simulink model "commhdlQPSKTxRxLoopback"  (R2025b)
settings: Solver=FixedStepDiscrete  StartTime=0.0  StopTime=stopTime  RelTol=1e-3
PostLoadFcn:
  | hScopeConfig = get_param([gcs '/Receiver/QPSK Rx/Frequency and Time Synchronizer/Symbol Synchronizer/No HDL/QPSK Receiver Eye Diagram'],'ScopeConfiguration');
  | 
  | hScopeConfig.OpenAtSimulationStart = false;
  | hScopeConfig.Visible = false;
  | SamplesPerSymbol = 4;
  | %UpsamplesRx = 1;
  | clear hScopeConfig
InitFcn:
  | commhdlQPSKTxRxModelInit;
  | % Rate bridge: ADRV9002/Jupiter radio runs at 15.36 MHz = 2x the 7.68 MHz
  | % (4 samples/symbol @ Rsym=1.92 MHz) the QPSK Rx requires. The deployed
  | % Receiver must downsample the ADC stream by 2. UpsamplesRx=1 fed the QPSK
  | % Rx 8 sps (2x-upsampled) and broke symbol sync / the loopback bit check.
  | UpsamplesRx = 1;   %% T8 RATE FIX: rail 15.36e6 == ADC bus rate,
  | %% no ingress decimation (was 2 when the rail sat on the 7.68e6 rung)
  | UpsamplesTx = 1;
  | clear simTimingOffset;
StopFcn:
  | if exist('simTimingOffset','var')
  |   disp('Simulation completed');
  |   %QPSKTxRxVerification;
  | end
values from neighbouring files (symbols this model uses):
  Config = commhdlQPSKTxRxParameters    [commhdlQPSKTxRxModelInit.m]
  Rsym = eval(get_param(qpskFindTxInputData(gcs),'Rsym'))    [commhdlQPSKTxRxModelInit.m]
undefined symbols (not defined in the file or in its folder): Add, fsym, randsrc, RandStream, Shift
libraries: hdlsllib x143, simulink x45, dspsigops x34, dsphdlfiltering2 x6, dsphdlsigops2 x4, dsphdlmathfun2 x4, commdigbbndpm3 x4, dspmlti4 x2, commchan3 x1, commrflib2 x1, commcnvcod2 x1
(part 7 of 8)

== system commhdlQPSKTxRxLoopback/TxRxComposite/Receiver/QPSK Rx/Frequency and Time Synchronizer/Preamble Detector/FIFO/Validate Input Push Pop ==
  rst : Inport
  push : Inport  Port=2
  pop : Inport  Port=3
  Compare To Constant : hdlsllib/Logic and Bit Operations/Compare To Constant  relop===  const=0  OutDataTypeStr=boolean
  Compare To Constant1 : hdlsllib/Logic and Bit Operations/Compare To Constant  relop===  const=fifoSize  OutDataTypeStr=boolean
  Constant : Constant  Value=true  SampleTime=-1
  Constant1 : Constant  Value=false  SampleTime=-1
  Delay : Delay  DelayLength=1
  Logical Operator1 : Logic  Operator=XOR  AllPortsSameDT=off  OutDataTypeStr=boolean
  Logical Operator2 : Logic  Operator=NOT  AllPortsSameDT=off  OutDataTypeStr=boolean
  Logical Operator{3..5,7,9} (5 alike) : Logic  AllPortsSameDT=off  OutDataTypeStr=boolean
  Logical Operator6 : Logic  Operator=NOT  AllPortsSameDT=off  OutDataTypeStr=boolean
  Logical Operator8 : Logic  Operator=NOT  AllPortsSameDT=off  OutDataTypeStr=boolean
  MATLAB Function : MATLAB Function  TreatAsAtomicUnit=on  mask{initVal=0, countToVal=fifoSize}
      mask prompts: initVal "Initial value:"; countToVal "Count to value:"
  No HDL : Subsystem
  Switch : Switch  Criteria=u2 ~= 0  SaturateOnIntegerOverflow=off  InputSameDT=off
  valid push : Outport
  valid pop : Outport  Port=2
  numEntries : Outport  Port=3
  wires:
  Delay/1 -> Compare To Constant/1, numEntries/1, Compare To Constant1/1
  rst/1 -> MATLAB Function/1(rst)
  Compare To Constant/1 -> Logical Operator3/1
  pop/1 -> Logical Operator7/1, Logical Operator3/2
  Switch/1 -> MATLAB Function/3(dir)
  MATLAB Function/1(count) -> Delay/1
  Constant1/1 -> Switch/1
  Logical Operator3/1 -> Logical Operator6/1, No HDL/2(popEmptyFIFO)  "pop on empty FIFO"
  Logical Operator4/1 -> Logical Operator2/1, No HDL/1(pushFullFIFO)  "push on full FIFO"
  Constant/1 -> Switch/3
  Compare To Constant1/1 -> Logical Operator4/2
  Logical Operator7/1 -> Logical Operator1/2, Logical Operator8/1, valid pop/1, Switch/2
  Logical Operator6/1 -> Logical Operator7/2
  Logical Operator1/1 -> MATLAB Function/2(enb)
  push/1 -> Logical Operator9/1, Logical Operator5/1
  Logical Operator8/1 -> Logical Operator5/2
  Logical Operator5/1 -> Logical Operator4/1
  Logical Operator2/1 -> Logical Operator9/2
  Logical Operator9/1 -> valid push/1, Logical Operator1/1

== system commhdlQPSKTxRxLoopback/TxRxComposite/Receiver/QPSK Rx/Frequency and Time Synchronizer/Preamble Detector/Timing Adjust/No HDL ==
  note: This subsystem generates variables required for QPSKRxVerification for validation
  validIn : Inport
  timingOffset : Inport  Port=2
  syncPulse : Inport  Port=3
  Compare To Constant : simulink/Logic and Bit Operations/Compare To Constant  relop===  const=0  OutDataTypeStr=boolean
  Delay : Delay  DelayLength=4
  Delay1 : Delay  DelayLength=4
  Frame Counter : hdlsllib/Sources/HDL Counter  CountType=Free running  CountInit=0  CountStep=1  CountMax=bitsPerPacket/2 - 1  CountFromType=Initial value  CountFrom=0  CountResetPort=off  CountLoadPort=off  CountEnbPort=on  CountDirPort=off  CountHitOutputPort=off  CountDataType=Unsigned  CountWordLen=32  CountFracLen=0  CountSampTime=1
  Logical Operator : Logic  AllPortsSameDT=off  OutDataTypeStr=boolean
  No HDL : Subsystem
  No HDL1 : Subsystem
  Symbol Counter : hdlsllib/Sources/HDL Counter  CountType=Count limited  CountInit=0  CountStep=1  CountMax=bitsPerPacket/2 - 1  CountFromType=Initial value  CountFrom=0  CountResetPort=off  CountLoadPort=off  CountEnbPort=on  CountDirPort=off  CountHitOutputPort=off  CountDataType=Unsigned  CountWordLen=nextpow2(bitsPerPacket/2 - 1)  CountFracLen=0  CountSampTime=1
  Unit Delay Enabled Synchronous : hdlsllib/Discrete/Unit Delay Enabled Synchronous  InitialCondition=0.0  SampleTime=-1
  wires:
  Delay1/1 -> No HDL/1(timingOffset)
  Delay/1 -> No HDL1/Enable, No HDL/Enable
  Unit Delay Enabled Synchronous/1 -> No HDL1/1(frameNumber)
  syncPulse/1 -> Delay/1
  Frame Counter/1 -> Unit Delay Enabled Synchronous/1
  Compare To Constant/1 -> Logical Operator/1
  Logical Operator/1 -> Frame Counter/1, Unit Delay Enabled Synchronous/2
  Symbol Counter/1 -> Compare To Constant/1
  validIn/1 -> Symbol Counter/1, Logical Operator/2
  timingOffset/1 -> Delay1/1

== system commhdlQPSKTxRxLoopback/TxRxComposite/Receiver/QPSK Rx/Frequency and Time Synchronizer/Symbol Synchronizer/Gardner TED/GTED ==
  In1 : Inport
  Add : Sum
  Add1 : Sum  Inputs=+-
  Add2 : Sum  Inputs=+-
  Complex to Real-Imag : ComplexToRealImag
  Delay{,1,4..5} (4 alike) : Delay  DelayLength=1
  Delay{9..10,12..13} (4 alike) : Delay
  Delay11 : Delay  DelayLength=4
  Delay{2..3,6..7} (4 alike) : Delay  DelayLength=3
  Delay8 : Delay  DelayLength=4
  Product : Product
  Product1 : Product
  Out1 : Outport
  wires:
  Delay13/1 -> Add/2
  Delay12/1 -> Product1/2
  Delay11/1 -> Product1/1
  Delay10/1 -> Add/1
  Delay9/1 -> Product/2
  Delay8/1 -> Product/1
  Complex to Real-Imag/2 -> Delay4/1, Add2/2
  Delay7/1 -> Add2/1
  Delay4/1 -> Delay5/1
  Delay6/1 -> Delay7/1
  Add2/1 -> Delay12/1
  Delay5/1 -> Delay6/1, Delay11/1
  Delay1/1 -> Delay8/1, Delay2/1
  Add1/1 -> Delay9/1
  Delay2/1 -> Delay3/1
  Delay/1 -> Delay1/1
  Delay3/1 -> Add1/1
  Complex to Real-Imag/1 -> Delay/1, Add1/2
  In1/1 -> Complex to Real-Imag/1
  Add/1 -> Out1/1
  Product1/1 -> Delay13/1
  Product/1 -> Delay10/1

== system commhdlQPSKTxRxLoopback/TxRxComposite/Receiver/QPSK Rx/Frequency and Time Synchronizer/Symbol Synchronizer/No HDL/No HDL ==
  data : Inport
  Enable : EnablePort
  Data Type Conversion : DataTypeConversion  OutDataTypeStr=double  SaturateOnIntegerOverflow=off  RndMeth=Floor
  wires:
  data/1 -> Data Type Conversion/1
  Data Type Conversion/1 -> ?

== system commhdlQPSKTxRxLoopback/TxRxComposite/Receiver/QPSK Rx/Frequency and Time Synchronizer/Symbol Synchronizer/Rate Handle/FIFO ==
  in : Inport
  push : Inport  Port=2
  pop : Inport  Port=3
  reset : Inport  Port=4
  Delay1 : Delay  DelayLength=1
  Pop Counter : hdlsllib/Sources/HDL Counter  CountType=Count limited  CountInit=0  CountStep=1  CountMax=fifoSize -1  CountFromType=Initial value  CountFrom=0  CountResetPort=on  CountLoadPort=off  CountEnbPort=on  CountDirPort=off  CountHitOutputPort=off  CountDataType=Unsigned  CountWordLen=nextpow2(fifoSize)  CountFracLen=0  CountSampTime=1
  Push Counter : hdlsllib/Sources/HDL Counter  CountType=Count limited  CountInit=0  CountStep=1  CountMax=fifoSize -1  CountFromType=Initial value  CountFrom=0  CountResetPort=on  CountLoadPort=off  CountEnbPort=on  CountDirPort=off  CountHitOutputPort=off  CountDataType=Unsigned  CountWordLen=nextpow2(fifoSize)  CountFracLen=0  CountSampTime=1
  Simple Dual Port RAM : hdlsllib/HDL RAMs/Simple Dual Port RAM  ram_size=nextpow2(fifoSize)
  Validate Input Push Pop : Subsystem
  out : Outport
  numEntries : Outport  Port=2
  validPop : Outport  Port=3
  wires:
  Validate Input Push Pop/3(numEntries) -> numEntries/1
  Simple Dual Port RAM/1 -> out/1
  Push Counter/1 -> Simple Dual Port RAM/2
  Pop Counter/1 -> Simple Dual Port RAM/4
  push/1 -> Validate Input Push Pop/2(push)
  pop/1 -> Validate Input Push Pop/3(pop)
  Validate Input Push Pop/1(valid push) -> Simple Dual Port RAM/3, Push Counter/2
  Validate Input Push Pop/2(valid pop) -> validPop/1, Pop Counter/2
  reset/1 -> Delay1/1, Validate Input Push Pop/1(rst)
  in/1 -> Simple Dual Port RAM/1
  Delay1/1 -> Pop Counter/1, Push Counter/1

== system commhdlQPSKTxRxLoopback/TxRxComposite/Transmitter/QPSK Tx/Bit Packetizer/Data Bits FIFO/No HDL/No HDL ==
  push : Inport
  full : Inport  Port=2
  ncount : Inport  Port=3
  empty : Inport  Port=4
  pop : Inport  Port=5
  Assertion : Assertion
  Assertion1 : Assertion
  Display : Display
  Logical Operator : Logic  Operator=NAND  AllPortsSameDT=off  OutDataTypeStr=boolean
  Logical Operator1 : Logic  Operator=NAND  AllPortsSameDT=off  OutDataTypeStr=boolean
  wires:
  push/1 -> Logical Operator/1
  empty/1 -> Logical Operator1/1
  full/1 -> Logical Operator/2
  pop/1 -> Logical Operator1/2
  Logical Operator/1 -> Assertion/1
  ncount/1 -> Display/1
  Logical Operator1/1 -> Assertion1/1

== system commhdlQPSKTxRxLoopback/Receiver/QPSK Rx/Frequency and Time Synchronizer/Symbol Synchronizer/Rate Handle/FIFO/Validate Input Push Pop/No HDL ==
  pushFullFIFO : Inport
  popEmptyFIFO : Inport  Port=2
  Constant2 : Constant  Value=pushFullDiag  SampleTime=-1
  Constant3 : Constant  Value=popEmptyDiag  SampleTime=-1
  MATLAB Function : MATLAB Function  TreatAsAtomicUnit=on
  wires:
  Constant2/1 -> MATLAB Function/1(pushFullDiag)
  Constant3/1 -> MATLAB Function/2(popEmptyDiag)
  popEmptyFIFO/1 -> MATLAB Function/4(popEmpty)
  pushFullFIFO/1 -> MATLAB Function/3(pushFull)

== system commhdlQPSKTxRxLoopback/TxRxComposite/Receiver/QPSK Rx/Frequency and Time Synchronizer/Coarse Frequency Compensator/Coarse Frequency Estimator/Integrator/Reset Generator ==
  validIn : Inport
  Compare To Constant : simulink/Logic and Bit Operations/Compare To Constant  relop===  const=integAvgLen  OutDataTypeStr=boolean
  Delay1 : Delay  DelayLength=1
  Delay5 : Delay  DelayLength=1
  HDL Counter : hdlsllib/Sources/HDL Counter  CountType=Count limited  CountInit=0  CountStep=1  CountMax=integAvgLen  CountFromType=Initial value  CountFrom=0  CountResetPort=off  CountLoadPort=off  CountEnbPort=on  CountDirPort=off  CountHitOutputPort=off  CountDataType=Unsigned  CountWordLen=nextpow2(integAvgLen + 1)  CountFracLen=0  CountSampTime=1
  Logical Operator : Logic  AllPortsSameDT=off  OutDataTypeStr=boolean
  reset : Outport
  wires:
  HDL Counter/1 -> Delay5/1
  Compare To Constant/1 -> Logical Operator/2
  validIn/1 -> Delay1/1, HDL Counter/1
  Logical Operator/1 -> reset/1
  Delay5/1 -> Compare To Constant/1
  Delay1/1 -> Logical Operator/1

== system commhdlQPSKTxRxLoopback/TxRxComposite/Receiver/QPSK Rx/Frequency and Time Synchronizer/Phase Ambiguity Estimation and Correction/Phase Ambiguity Corrector/Reciprocal/Function Impl ==
  switch : Inport
  LUTAddr : Inport  Port=2
  Delay{6..8,10,15..16} (6 alike) : Delay
  Delay9 : Delay  DelayLength=1
  LUT1 : LookupNDDirect  NumberOfTableDimensions=1  Table=LUT(:,1)  DiagnosticForOutOfRangeInput=Error
  LUT2 : LookupNDDirect  NumberOfTableDimensions=1  Table=LUT(:,2)  DiagnosticForOutOfRangeInput=Error
  Multiport Switch : MultiPortSwitch  DataPortOrder=Zero-based contiguous  Inputs=2  zeroidx=on  SaturateOnIntegerOverflow=off  InputSameDT=off
  functionValues : Outport
  wires:
  LUTAddr/1 -> Delay7/1, Delay6/1
  Delay15/1 -> Multiport Switch/2
  Delay16/1 -> Multiport Switch/3
  Delay10/1 -> Multiport Switch/1
  Delay9/1 -> functionValues/1
  LUT2/1 -> Delay15/1
  LUT1/1 -> Delay16/1
  switch/1 -> Delay8/1
  Delay8/1 -> Delay10/1
  Delay7/1 -> LUT2/1
  Delay6/1 -> LUT1/1
  Multiport Switch/1 -> Delay9/1

== system commhdlQPSKTxRxLoopback/TxRxComposite/Receiver/QPSK Rx/Frequency and Time Synchronizer/Preamble Detector/FIFO/Validate Input Push Pop/No HDL ==
  pushFullFIFO : Inport
  popEmptyFIFO : Inport  Port=2
  Constant2 : Constant  Value=pushFullDiag  SampleTime=-1
  Constant3 : Constant  Value=popEmptyDiag  SampleTime=-1
  MATLAB Function : MATLAB Function  TreatAsAtomicUnit=on
  wires:
  pushFullFIFO/1 -> MATLAB Function/3(pushFull)
  popEmptyFIFO/1 -> MATLAB Function/4(popEmpty)
  Constant3/1 -> MATLAB Function/2(popEmptyDiag)
  Constant2/1 -> MATLAB Function/1(pushFullDiag)

== system commhdlQPSKTxRxLoopback/TxRxComposite/Receiver/QPSK Rx/Frequency and Time Synchronizer/Preamble Detector/Timing Adjust/No HDL/No HDL ==
  timingOffset : Inport
  Enable : EnablePort
  Data Type Conversion : DataTypeConversion  OutDataTypeStr=double  SaturateOnIntegerOverflow=off  RndMeth=Floor
  wires:
  timingOffset/1 -> Data Type Conversion/1
  Data Type Conversion/1 -> ?

== system commhdlQPSKTxRxLoopback/TxRxComposite/Receiver/QPSK Rx/Frequency and Time Synchronizer/Preamble Detector/Timing Adjust/No HDL/No HDL1 ==
  frameNumber : Inport
  Enable : EnablePort
  Data Type Conversion : DataTypeConversion  OutDataTypeStr=double  SaturateOnIntegerOverflow=off  RndMeth=Floor
  wires:
  Data Type Conversion/1 -> ?
  frameNumber/1 -> Data Type Conversion/1

== system commhdlQPSKTxRxLoopback/TxRxComposite/Receiver/QPSK Rx/Frequency and Time Synchronizer/Symbol Synchronizer/Rate Handle/FIFO/Validate Input Push Pop ==
  rst : Inport
  push : Inport  Port=2
  pop : Inport  Port=3
  Compare To Constant : hdlsllib/Logic and Bit Operations/Compare To Constant  relop===  const=0  OutDataTypeStr=boolean
  Compare To Constant1 : hdlsllib/Logic and Bit Operations/Compare To Constant  relop===  const=fifoSize  OutDataTypeStr=boolean
  Constant : Constant  Value=true  SampleTime=-1
  Constant1 : Constant  Value=false  SampleTime=-1
  Delay : Delay  DelayLength=1
  Logical Operator1 : Logic  Operator=XOR  AllPortsSameDT=off  OutDataTypeStr=boolean
  Logical Operator2 : Logic  Operator=NOT  AllPortsSameDT=off  OutDataTypeStr=boolean
  Logical Operator{3..5,7,9} (5 alike) : Logic  AllPortsSameDT=off  OutDataTypeStr=boolean
  Logical Operator6 : Logic  Operator=NOT  AllPortsSameDT=off  OutDataTypeStr=boolean
  Logical Operator8 : Logic  Operator=NOT  AllPortsSameDT=off  OutDataTypeStr=boolean
  MATLAB Function : MATLAB Function  TreatAsAtomicUnit=on  mask{initVal=0, countToVal=fifoSize}
      mask prompts: initVal "Initial value:"; countToVal "Count to value:"
  No HDL : Subsystem
  Switch : Switch  Criteria=u2 ~= 0  SaturateOnIntegerOverflow=off  InputSameDT=off
  valid push : Outport
  valid pop : Outport  Port=2
  numEntries : Outport  Port=3
  wires:
  Delay/1 -> Compare To Constant/1, numEntries/1, Compare To Constant1/1
  rst/1 -> MATLAB Function/1(rst)
  Compare To Constant/1 -> Logical Operator3/1
  pop/1 -> Logical Operator7/1, Logical Operator3/2
  Switch/1 -> MATLAB Function/3(dir)
  MATLAB Function/1(count) -> Delay/1
  Constant1/1 -> Switch/1
  Logical Operator3/1 -> Logical Operator6/1, No HDL/2(popEmptyFIFO)  "pop on empty FIFO"
  Logical Operator4/1 -> Logical Operator2/1, No HDL/1(pushFullFIFO)  "push on full FIFO"
  Constant/1 -> Switch/3
  Compare To Constant1/1 -> Logical Operator4/2
  Logical Operator7/1 -> Logical Operator1/2, Logical Operator8/1, valid pop/1, Switch/2
  Logical Operator6/1 -> Logical Operator7/2
  Logical Operator1/1 -> MATLAB Function/2(enb)
  push/1 -> Logical Operator9/1, Logical Operator5/1
  Logical Operator8/1 -> Logical Operator5/2
  Logical Operator5/1 -> Logical Operator4/1
  Logical Operator2/1 -> Logical Operator9/2
  Logical Operator9/1 -> valid push/1, Logical Operator1/1

== system commhdlQPSKTxRxLoopback/TxRxComposite/Receiver/QPSK Rx/Frequency and Time Synchronizer/Symbol Synchronizer/Rate Handle/FIFO/Validate Input Push Pop/No HDL ==
  pushFullFIFO : Inport
  popEmptyFIFO : Inport  Port=2
  Constant2 : Constant  Value=pushFullDiag  SampleTime=-1
  Constant3 : Constant  Value=popEmptyDiag  SampleTime=-1
  MATLAB Function : MATLAB Function  TreatAsAtomicUnit=on
  wires:
  pushFullFIFO/1 -> MATLAB Function/3(pushFull)
  popEmptyFIFO/1 -> MATLAB Function/4(popEmpty)
  Constant3/1 -> MATLAB Function/2(popEmptyDiag)
  Constant2/1 -> MATLAB Function/1(pushFullDiag)

== matlab function commhdlQPSKTxRxLoopback/Receiver/QPSK Rx/Frequency and Time Synchronizer/Symbol Synchronizer/Rate Handle/FIFO/Validate Input Push Pop/No HDL/MATLAB Function ==
  data: pushFullDiag input; popEmptyDiag input; pushFull input; popEmpty input
function pushPopDiagnostics(pushFullDiag, popEmptyDiag, pushFull, popEmpty)
%#codegen


if(pushFull)
    switch pushFullDiag
        case 2
            warning('Push signal applied on full FIFO');
        case 3
            error('Push signal applied on full FIFO');
        otherwise
    end
end

if(popEmpty)
    switch popEmptyDiag
        case 2
            warning('Pop signal applied on empty FIFO');
        case 3
            error('Pop signal applied on empty FIFO');
        otherwise
    end
end

end

== matlab function commhdlQPSKTxRxLoopback/Receiver/Capture Data Bits/MATLAB Function ==
  data: valid input; datain input; start input; stop input; count_out output; packets_out output; bit_errors_out output
function [count_out, packets_out, bit_errors_out] = msgdec(valid, datain, start, stop)

persistent count;
persistent msgbuffer;

persistent packetsReceived
persistent errors;

if isempty(count) || isempty(msgbuffer) || isempty(packetsReceived)
    count = uint32(0);
    msgbuffer = zeros(1,120+8)>0; % ADI Hello WorldX
    packetsReceived = uint32(0);
    errors = uint32(0);
end

% Mesg
strAscii = dec2bin('ADI Hello World',8);
msgarray = reshape(strAscii', [1, numel(strAscii)]);
msgbits = logical(msgarray - 48);

% msgLen = uint32(2240);

if valid
    if start
        count = uint32(1);
        packetsReceived = packetsReceived + 1;
    end

    if count <= (length(msgbuffer) - 8)
        msgbuffer(count) = datain;
        if datain ~= msgbits(count)
            errors = errors + 1;
        end

    elseif count == length(msgbuffer) + 1
        msgarray_dec = char('0' + msgbuffer);
        N = length(msgarray_dec) / 8;
        strAscii_dec = reshape(msgarray_dec , 8, N).';
        msg = char(bin2dec(strAscii_dec).');
        disp(msg);
    end
    
    if count <= length(msgbuffer) + 2
        count = count + 1;
    end
end

count_out = count;
packets_out = packetsReceived;
bit_errors_out = errors;

== matlab function commhdlQPSKTxRxLoopback/TxRxComposite/Transmitter/Input Data/Message Generator/MATLAB Function ==
  data: enable input; reset input; out output; start output; stop output; valid output; count_out output; msg_count_out output
function [out, start, stop, valid, count_out, msg_count_out] = msggen(enable, reset)

persistent indexCount;
persistent toggle;
persistent msgCount;
persistent msgCountAll;
persistent msgCountBitIndex;

if isempty(indexCount) || isempty(toggle) || isempty(msgCount) || isempty(msgCountBitIndex) || isempty(msgCountAll)
    indexCount = uint32(0);
    msgCount = uint32(1);
    msgCountAll = uint32(1);
    msgCountBitIndex = uint8(0);
    toggle = false;
end

%% Constants -- FIXED pre-coded K=5 packet ROM (rom_words_70_k5.txt, 2240 bits,
%% word w = bits[32w..32w+31] MSB-first). Stored as 70 x uint32 packed words
%% (a large inline logical literal crashes the Stateflow compiler),
%% unpacked into the 2240-element msgbits logical ROM and indexed with the
%% STOCK msgbits(indexCount+1) pattern. Replaces the stock 120-bit message ROM.
%% Content: K=5 [35 23] rate-1/2 coded info(1084)+tail(4) -> 2176 bits,
%% 136x16 block-interleaved (perm r*16+c), + 64-bit PN9 filler. The K=5 Rx
%% deint(perm c*136+r) + Viterbi(TB=25) recovers the 120-bit BIST message.
romWords = uint32([1204691830 3483708319 2883549788 1307975730 2302022013 2317836649 3978304949 752593182 1746968124 1349240209 3902614806 3574627500 2876326604 954122960 3619913623 992243276 1282392315 4164772487 4184517345 1152214674 4291480147 2890259028 3610356907 1974996972 98969832 2966137360 2073901288 1031243679 383809583 502821458 1907466333 3571684694 1914253232 2851552230 1013061234 1172847641 1490586163 2615211549 1975790333 2449786334 370176357 2032636540 3182658485 272185979 820521565 988977659 268086207 3618645391 1183606930 3738257601 3934953195 2068097708 1140472544 1215563522 1259455610 488066730 3594016596 2108810799 1154262029 1112597399 709494092 949055130 535665595 1873753487 233633426 2298642372 2539920837 2482285935 4286832407 839470801]);
msgbits = false(1,2240);
for w = 0:69
    wv = romWords(w+1);
    for bb = 0:31
        msgbits(w*32 + bb + 1) = bitget(wv, 32 - bb) ~= uint32(0);
    end
end
msgbitsLen = uint32(length(msgbits));

fullMessageLen = uint32(2240-1); %% Need the -1 to eat the feedback delay (stock hardcoded value in this model)

%% Logic
if enable && ~reset
    %% Set out data
    if indexCount < msgbitsLen %% Emit the fixed pre-coded packet bit (unpacked ROM)
        out = msgbits(indexCount + 1);
        msgCountBitIndex = uint8(0);
    else %% beyond the ROM (should not occur: msgbitsLen==dataBitsPerPacket)
        out = false;
        msgCountBitIndex = uint8(0);
    end

    %% Flags
    start = indexCount == uint32(0);
    stop = indexCount == fullMessageLen;
    valid = true;

    %% Counters
    if fullMessageLen == indexCount
        if msgCount >= 9
            msgCount = uint32(1);
        else
            msgCount = msgCount +  1;
            msgCountAll = msgCountAll + 1;
        end
    end
    if indexCount <= fullMessageLen
        indexCount = indexCount + 1;
    end

else %% Enable == false

    if reset
        indexCount = uint32(0);
        msgCountBitIndex = uint8(0);
        toggle = false;
    end
    out = false;
    start = false;
    stop = false;
    valid = false;
end

if isempty(indexCount)
    count_out = uint32(0);
else
    count_out = indexCount;
end

msg_count_out = msgCountAll;

== matlab function commhdlQPSKTxRxLoopback/Receiver/QPSK Rx/Frequency and Time Synchronizer/Preamble Detector/FIFO/Validate Input Push Pop/MATLAB Function ==
  data: rst input; count output; enb input; dir input; initVal parameter; countToVal parameter
function count = hdlCounter(rst,enb,dir,initVal,countToVal)
%#codegen

persistent countReg

if(isempty(countReg))
    countReg = fi(initVal,0,nextpow2(countToVal+1),0);
end

if(rst)
    countReg(:) = initVal;
elseif(enb)
    if(dir)
        if(countReg==countToVal)
            countReg(:) = initVal;
        else
            countReg(:) = countReg+1;
        end
    else
        if(countReg==initVal)
            countReg(:) = countToVal;
        else
            countReg(:) = countReg-1;
        end
    end
end

count = countReg;

end

== matlab function commhdlQPSKTxRxLoopback/Receiver/QPSK Rx/Frequency and Time Synchronizer/Preamble Detector/FIFO/Validate Input Push Pop/No HDL/MATLAB Function ==
  data: pushFullDiag input; popEmptyDiag input; pushFull input; popEmpty input
function pushPopDiagnostics(pushFullDiag, popEmptyDiag, pushFull, popEmpty)
%#codegen


if(pushFull)
    switch pushFullDiag
        case 2
            warning('Push signal applied on full FIFO');
        case 3
            error('Push signal applied on full FIFO');
        otherwise
    end
end

if(popEmpty)
    switch popEmptyDiag
        case 2
            warning('Pop signal applied on empty FIFO');
        case 3
            error('Pop signal applied on empty FIFO');
        otherwise
    end
end

end

== matlab function commhdlQPSKTxRxLoopback/TxRxComposite/Transmitter/QPSK Tx/Bit Packetizer/Data Bits FIFO/MATLAB Function1 ==
  data: wr input; full output; rd input; dataBitsPerPacket parameter
function full = fcn(wr,rd,dataBitsPerPacket)
%#codegen
     
    depth = dataBitsPerPacket*2 - 1;
    persistent count;
    if isempty(count)
        count = fi(0,0,nextpow2(depth),0,hdlfimath);
    end

    if wr
        count(:) = count + 1;
    end
    if rd
        count(:) = count - 1;
    end

    full = (count > depth);

end

== matlab function commhdlQPSKTxRxLoopback/Transmitter/QPSK Tx/Bit Packetizer/Data Bits FIFO/No HDL/MATLAB Function ==
  data: wr input; full output; rd input; ncount output; empty output; dataBitsPerPacket parameter
function [full,ncount,empty] = fcn(wr,rd,dataBitsPerPacket)
%#codegen
     
    depth = dataBitsPerPacket*2 - 1;
    persistent count;
    if isempty(count)
        count = fi(0,0,nextpow2(depth),0,hdlfimath);
    end

    empty = (count == 0);
    full = (count > depth);
    ncount = count;

    if wr
        count(:) = count + 1;
    end
    if rd
        count(:) = count - 1;
    end

end

== matlab function commhdlQPSKTxRxLoopback/TxRxComposite/Transmitter/QPSK Tx/Bit Packetizer/Data Bits FIFO/No HDL/MATLAB Function ==
  data: wr input; full output; rd input; ncount output; empty output; dataBitsPerPacket parameter
function [full,ncount,empty] = fcn(wr,rd,dataBitsPerPacket)
%#codegen
     
    depth = dataBitsPerPacket*2 - 1;
    persistent count;
    if isempty(count)
        count = fi(0,0,nextpow2(depth),0,hdlfimath);
    end

    empty = (count == 0);
    full = (count > depth);
    ncount = count;

    if wr
        count(:) = count + 1;
    end
    if rd
        count(:) = count - 1;
    end

end

== matlab function commhdlQPSKTxRxLoopback/TxRxComposite/Transmitter/QPSK Tx/Bit Packetizer/Data Bits FIFO/RAM Frame Status Indicator ==
  data: push input; out output; pop input; dataBitsPerPacket parameter
function out = fcn(push,pop,dataBitsPerPacket)

   persistent pushCount popCount frameCount;
   if isempty(pushCount)
       pushCount = fi(0,0,nextpow2(dataBitsPerPacket),0,hdlfimath);
       frameCount = fi(0,0,2,0,hdlfimath);
       popCount = fi(0,0,nextpow2(dataBitsPerPacket),0,hdlfimath);
   end
   
   if (pushCount == dataBitsPerPacket-1) && push
       frameCount(:) = frameCount + 1;
   end
   if (popCount == dataBitsPerPacket-1) && pop
       frameCount(:) = frameCount - 1;
   end

   if push
       if pushCount == dataBitsPerPacket - 1
           pushCount(:) = 0;
       else
           pushCount(:) = pushCount + 1;
       end
   end

   if pop 
       if popCount == dataBitsPerPacket - 1
           popCount(:) = 0;
       else
           popCount(:) = popCount + 1;
       end
   end

   out = frameCount;

end

== matlab function commhdlQPSKTxRxLoopback/TxRxComposite/Receiver/Capture Data Bits/MATLAB Function ==
  data: valid input; datain input; start input; stop input; count_out output; packets_out output; bit_errors_out output
function [count_out, packets_out, bit_errors_out] = msgdec(valid, datain, start, stop)

persistent count;
persistent msgbuffer;

persistent packetsReceived
persistent errors;

if isempty(count) || isempty(msgbuffer) || isempty(packetsReceived)
    count = uint32(0);
    msgbuffer = zeros(1,120+8)>0; % ADI Hello WorldX
    packetsReceived = uint32(0);
    errors = uint32(0);
end

% Mesg
strAscii = dec2bin('ADI Hello World',8);
msgarray = reshape(strAscii', [1, numel(strAscii)]);
msgbits = logical(msgarray - 48);

% msgLen = uint32(2240);

if valid
    if start
        count = uint32(1);
        packetsReceived = packetsReceived + 1;
    end

    if count <= (length(msgbuffer) - 8)
        msgbuffer(count) = datain;
        if datain ~= msgbits(count)
            errors = errors + 1;
        end

    elseif count == length(msgbuffer) + 1
        msgarray_dec = char('0' + msgbuffer);
        N = length(msgarray_dec) / 8;
        strAscii_dec = reshape(msgarray_dec , 8, N).';
        msg = char(bin2dec(strAscii_dec).');
        disp(msg);
    end
    
    if count <= length(msgbuffer) + 2
        count = count + 1;
    end
end

count_out = count;
packets_out = packetsReceived;
bit_errors_out = errors;

== matlab function commhdlQPSKTxRxLoopback/TxRxComposite/Receiver/QPSK Rx/Frequency and Time Synchronizer/Packet Controller/MATLAB Function ==
  data: valid input; syncPulse input; out output
function out = fcn(valid,syncPulse)
%#codegen

  persistent Reg;
  if isempty(Reg)
      Reg = false;
  end
  
  out = Reg;
  
  if Reg && valid
      Reg = false;
  end
  
  if syncPulse
      Reg = true;
  end
  
end

== matlab function commhdlQPSKTxRxLoopback/TxRxComposite/Receiver/QPSK Rx/Frequency and Time Synchronizer/Packet Controller/sample discard controller ==
  data: dataIn input; validIn input; dataOut output; startIn input; endIn input; startOut output; endOut output; validOut output
function [dataOut,startOut,endOut,validOut] = controller(dataIn,validIn,startIn,endIn)
%#codegen

   persistent active dataOutReg validOutReg startOutReg endOutReg;
   if isempty(active)
      active  = false;
      dataOutReg = cast(0,'like',dataIn);
      validOutReg = false;
      startOutReg = false;
      endOutReg = false;
   end
   
   dataOut = dataOutReg;
   validOut = validOutReg;
   startOut = startOutReg;
   endOut = endOutReg;
   
   startOutReg = startIn;
   endOutReg = endIn;
   
   if startIn
       active = true;
   end
   
   if active
       dataOutReg(:) = dataIn;
       validOutReg = validIn;
   else
       dataOutReg(:) = 0;
       validOutReg = false;
   end
   
   if endIn
       if active 
           endOutReg = true;
       else
           endOutReg = false;
       end
       active = false;
   end
end

== matlab function commhdlQPSKTxRxLoopback/TxRxComposite/Receiver/QPSK Rx/Frequency and Time Synchronizer/Preamble Detector/Correlator/ThresholdLimiter ==
  settings: fimath=hdlfimath
  data: x input; y output
function y = applyLowerLimit(x)
    % Apply a lower limit to the threshold.
    %#codegen
    
    % Threshold is computed by summing across 63 samples.
    % Set lower limit to be equivalent of all 63 samples
    % having their LSB set to 1 and all others set to 0. 
    lowerLimit = cast(0.01, 'like', x);
    
    if x < lowerLimit
        y = lowerLimit;
    else
        y = x;
    end
end

== matlab function commhdlQPSKTxRxLoopback/TxRxComposite/Receiver/QPSK Rx/Frequency and Time Synchronizer/Preamble Detector/FIFO/Validate Input Push Pop/MATLAB Function ==
  data: rst input; count output; enb input; dir input; initVal parameter; countToVal parameter
function count = hdlCounter(rst,enb,dir,initVal,countToVal)
%#codegen

persistent countReg

if(isempty(countReg))
    countReg = fi(initVal,0,nextpow2(countToVal+1),0);
end

if(rst)
    countReg(:) = initVal;
elseif(enb)
    if(dir)
        if(countReg==countToVal)
            countReg(:) = initVal;
        else
            countReg(:) = countReg+1;
        end
    else
        if(countReg==initVal)
            countReg(:) = countToVal;
        else
            countReg(:) = countReg-1;
        end
    end
end

count = countReg;

end

== matlab function commhdlQPSKTxRxLoopback/TxRxComposite/Receiver/QPSK Rx/Frequency and Time Synchronizer/Preamble Detector/FIFO/Validate Input Push Pop/No HDL/MATLAB Function ==
  data: pushFullDiag input; popEmptyDiag input; pushFull input; popEmpty input
function pushPopDiagnostics(pushFullDiag, popEmptyDiag, pushFull, popEmpty)
%#codegen


if(pushFull)
    switch pushFullDiag
        case 2
            warning('Push signal applied on full FIFO');
        case 3
            error('Push signal applied on full FIFO');
        otherwise
    end
end

if(popEmpty)
    switch popEmptyDiag
        case 2
            warning('Pop signal applied on empty FIFO');
        case 3
            error('Pop signal applied on empty FIFO');
        otherwise
    end
end

end

== matlab function commhdlQPSKTxRxLoopback/Receiver/QPSK Rx/Frequency and Time Synchronizer/Packet Controller/MATLAB Function ==
  data: valid input; syncPulse input; out output
function out = fcn(valid,syncPulse)
%#codegen

  persistent Reg;
  if isempty(Reg)
      Reg = false;
  end
  
  out = Reg;
  
  if Reg && valid
      Reg = false;
  end
  
  if syncPulse
      Reg = true;
  end
  
end

== matlab function commhdlQPSKTxRxLoopback/TxRxComposite/Receiver/QPSK Rx/Frequency and Time Synchronizer/Symbol Synchronizer/Interpolation Control ==
  data: mu output; Delta input; Underflow output; stateWord output
function [mu,Underflow,stateWord] = Interpolation_ctrl(Delta)
% Implementation of modulo-1 counter for interpolation control listed in
% Figure 8.4.19 of "Digital Communications - A Discrete-Time Approach"
% by Michael Rice. See design details in Chapter 8.4.3 of the same book.
% 
% Input:
%   Delta - Loop filter output. If loop is in lock, delta would be small
% Output:
%   Underflow - Indicator of counter underflow. This is the strobe signal
%               for downstream processing
%   mu - Difference between actual sampling instant and the optimal instant,
%        between zero and one
%#codegen

% countReg - Counter value delayed by 1 sample
% muReg - The estimated timing error normalized by half QPSK symbols

   mask = fi(1-2^(-10),1,11,10);
   
   persistent countReg underflowReg muReg;
   if isempty(countReg)
       countReg  = fi(0,1,11,10);
       muReg = fi(0,1,11,10);
       underflowReg = false;
   end
   
   
   Underflow = underflowReg;
   % T8.7 telemetry: {und[22] | countReg[21:11] | mu[10:0]} stored-int
   stateWord = bitor(bitor(uint32(reinterpretcast(muReg, numerictype(0,11,0))), ...
       bitshift(uint32(reinterpretcast(countReg, numerictype(0,11,0))), 11)), ...
       bitshift(uint32(underflowReg), 22));

   mu = muReg;   
   
   
      % T8.4 anti-wedge clamp: if Delta <= -0.125 the decrementing counter
   % never underflows (strobes stop FOREVER -- Class-4 wedge / Class-1
   % episode mechanism; see tb_timing_wedge.v). Bound Delta so the
   % counter always decrements by >= 1 LSB.
   wlim = fi(127/1024,1,11,10);
   if Delta > wlim
       Delta = wlim;
   elseif Delta < -wlim
       Delta = fi(-127/1024,1,11,10);
   end
   counter = bitand(mask,countReg)-Delta-fi(0.125,1,11,10); % decrementing counter
   
   % if countReg is a nonnegative number,
   % then mod(countReg,1) equals the fractional part of countReg
   if counter < 0
       underflowReg = true;
       muReg = bitshift(bitand(mask,countReg),3);
       countReg = fi(counter+1,1,11,10);% create underflow to counter
   else
       underflowReg = false;
       countReg = fi(counter,1,11,10);
   end
   


end

== matlab function commhdlQPSKTxRxLoopback/TxRxComposite/Receiver/QPSK Rx/Frequency and Time Synchronizer/Symbol Synchronizer/Rate Handle/FIFO/Validate Input Push Pop/MATLAB Function ==
  data: rst input; count output; enb input; dir input; initVal parameter; countToVal parameter
function count = hdlCounter(rst,enb,dir,initVal,countToVal)
%#codegen

persistent countReg

if(isempty(countReg))
    countReg = fi(initVal,0,nextpow2(countToVal+1),0);
end

if(rst)
    countReg(:) = initVal;
elseif(enb)
    if(dir)
        if(countReg==countToVal)
            countReg(:) = initVal;
        else
            countReg(:) = countReg+1;
        end
    else
        if(countReg==initVal)
            countReg(:) = countToVal;
        else
            countReg(:) = countReg-1;
        end
    end
end

count = countReg;

end

== matlab function commhdlQPSKTxRxLoopback/TxRxComposite/Receiver/QPSK Rx/Frequency and Time Synchronizer/Symbol Synchronizer/Rate Handle/FIFO/Validate Input Push Pop/No HDL/MATLAB Function ==
  data: pushFullDiag input; popEmptyDiag input; pushFull input; popEmpty input
function pushPopDiagnostics(pushFullDiag, popEmptyDiag, pushFull, popEmpty)
%#codegen


if(pushFull)
    switch pushFullDiag
        case 2
            warning('Push signal applied on full FIFO');
        case 3
            error('Push signal applied on full FIFO');
        otherwise
    end
end

if(popEmpty)
    switch popEmptyDiag
        case 2
            warning('Pop signal applied on empty FIFO');
        case 3
            error('Pop signal applied on empty FIFO');
        otherwise
    end
end

end

== matlab function commhdlQPSKTxRxLoopback/TxRxComposite/Receiver/QPSK Rx/FEC Decoder Wrapper/RxDeint ==
  data: dataIn input; codedPair output; startIn input; endIn input; validIn input; vitReset output; deintValid output; frameStart output; frameEnd output; setIn input; clrIn input
function [codedPair, vitReset, deintValid, frameStart, frameEnd] = fecRxDeint(dataIn, startIn, endIn, validIn, setIn, clrIn)
%#codegen
persistent ramA ramB rdBank wptr pcnt hold0 hold1 rdGate rcol rrow skipCnt pendD;
CODED=uint16(2176); COLS=uint16(16); ROWS=uint16(136);
NPAIR=uint16(1088);
if isempty(ramA), ramA=false(1,2176); ramB=false(1,2176); rdBank=false; wptr=uint16(0); pcnt=uint16(0); hold0=false; hold1=false; rdGate=false; rcol=uint16(0); rrow=uint16(0); skipCnt=uint16(0); pendD=false; end
rb=rdBank; w=wptr; pc=pcnt; g=rdGate; h0=hold0; h1=hold1; cc=rcol; rr=rrow;
skc=skipCnt; pend=(pendD || logical(setIn)) && ~logical(clrIn);
pair0=h0; pair1=h1;
vitReset=false; deintValid=false; frameStart=false; frameEnd=false;
wrPos=uint16(65535); wrBit=false; wrBankA=false; doWr=false;
if validIn
  if startIn, w=uint16(0); pc=uint16(0); rb=~rb; g=true; cc=uint16(0); rr=uint16(0); if pend, skc=uint16(64); pend=false; else, skc=uint16(0); end, end % rdGate=TRUE: frame pair0 read COINCIDES with frameStart (RxAlign arms on that beat); read-counters reset in lockstep with pc
  % ---- READ side first (opposite bank; RXROOT E8 isolated reads: 1 pair per 2 validIn beats) ----
  if g && (pc < NPAIR)
    % divisionless read address: cc (even col) / rr (row) are incremental counters.
    % rc0=2*pc is even so rc1=rc0+1 keeps the same row -> perm1 = perm0 + ROWS (one add).
    perm0 = cc*ROWS + rr;
    perm1 = perm0 + ROWS;
    b0v = false; b1v = false;
    if perm0 < CODED
      if rb, b0v = ramB(double(perm0)+1); else b0v = ramA(double(perm0)+1); end
    end
    if perm1 < CODED
      if rb, b1v = ramB(double(perm1)+1); else b1v = ramA(double(perm1)+1); end
    end
    pair0 = b0v; pair1 = b1v; h0 = b0v; h1 = b1v;
    deintValid = true;
    if pc == uint16(0), vitReset = true; end
    pc = pc + 1;
    cc = cc + uint16(2);
    if cc == COLS, cc = uint16(0); rr = rr + uint16(1); end
  end
  % ---- WRITE side after all reads ----
  if skc > uint16(0)
    skc = skc - uint16(1);
  elseif w < CODED
    wrPos = w; wrBit = logical(dataIn); wrBankA = rb; doWr = true;
    w = w + 1;
  end
  g = ~g;
  frameStart=startIn; frameEnd=endIn;
end
codedPair = fi([pair0; pair1], 0, 1, 0);
% ---- persist state last ----
if doWr
  if wrBankA, ramA(double(wrPos)+1)=wrBit; else ramB(double(wrPos)+1)=wrBit; end
end
rdBank=rb; wptr=w; pcnt=pc; rdGate=g; hold0=h0; hold1=h1; rcol=cc; rrow=rr; skipCnt=skc; pendD=pend;

== matlab function commhdlQPSKTxRxLoopback/TxRxComposite/Receiver/QPSK Rx/FEC Decoder Wrapper/RxAlign ==
  data: decBit input; dataOut output; deintValid input; frameStart input; frameEnd input; skipCount input; startOut output; endOut output; validOut output
function [dataOut, startOut, endOut, validOut] = fecRxAlign(decBit, deintValid, frameStart, frameEnd, skipCount)
%#codegen
persistent oc started skip;
INFO=uint16(1084);
if isempty(oc), oc=uint16(0); started=false; skip=uint16(0); end
o=oc; st=started; sk=skip;
dataOut=false; startOut=false; endOut=false; validOut=false;
sc = uint16(skipCount);
if sc > INFO, sc = INFO; end
if deintValid
  if frameStart, o=uint16(0); st=true; sk=sc+uint16(41); end % +41 = gated-Viterbi latency in deintValid beats incl. VitGate hold reg (RXROOT E8)
  if st
    if sk > uint16(0)
      sk = sk - uint16(1);
    elseif o < INFO
      dataOut = decBit;
      startOut = (o==uint16(0));
      endOut   = (o==(INFO-1));
      validOut = true;
      o = o + uint16(1);
    end
  end
end
oc=o; started=st; skip=sk;

== matlab function commhdlQPSKTxRxLoopback/TxRxComposite/Receiver/QPSK Rx/FEC Decoder Wrapper/FecCounters ==
  data: e1 input; c1 output; e2 input; e3 input; e4 input; e5 input; e6 input; c2 output; c3 output; c4 output; c5 output; c6 output
function [c1, c2, c3, c4, c5, c6] = fecCounters(e1, e2, e3, e4, e5, e6)
%#codegen
% Free-running FEC-Rx datapath event counters (reset by modem soft-reset 0x000).
persistent k1 k2 k3 k4 k5 k6;
if isempty(k1)
  k1=uint32(0); k2=uint32(0); k3=uint32(0); k4=uint32(0); k5=uint32(0); k6=uint32(0);
end
MAX=uint32(4294967295);
n1=k1; n2=k2; n3=k3; n4=k4; n5=k5; n6=k6;
if e1 && n1<MAX, n1=n1+uint32(1); end
if e2 && n2<MAX, n2=n2+uint32(1); end
if e3 && n3<MAX, n3=n3+uint32(1); end
if e4 && n4<MAX, n4=n4+uint32(1); end
if e5 && n5<MAX, n5=n5+uint32(1); end
if e6 && n6<MAX, n6=n6+uint32(1); end
c1=n1; c2=n2; c3=n3; c4=n4; c5=n5; c6=n6;
k1=n1; k2=n2; k3=n3; k4=n4; k5=n5; k6=n6;

== matlab function commhdlQPSKTxRxLoopback/Receiver/QPSK Rx/Frequency and Time Synchronizer/Symbol Synchronizer/Rate Handle/FIFO/Validate Input Push Pop/MATLAB Function ==
  data: rst input; count output; enb input; dir input; initVal parameter; countToVal parameter
function count = hdlCounter(rst,enb,dir,initVal,countToVal)
%#codegen

persistent countReg

if(isempty(countReg))
    countReg = fi(initVal,0,nextpow2(countToVal+1),0);
end

if(rst)
    countReg(:) = initVal;
elseif(enb)
    if(dir)
        if(countReg==countToVal)
            countReg(:) = initVal;
        else
            countReg(:) = countReg+1;
        end
    else
        if(countReg==initVal)
            countReg(:) = countToVal;
        else
            countReg(:) = countReg-1;
        end
    end
end

count = countReg;

end

== matlab function commhdlQPSKTxRxLoopback/TxRxComposite/Receiver/QPSK Rx/FEC Decoder Wrapper/FecCapture ==
  data: bitsIn input; capIn output; validIn input; startIn input; codedPair input; deintValid input; decBit input; skipCount input; outValid input; capDeint output; capOut output
function [capIn, capDeint, capOut] = fecCapture(bitsIn, validIn, startIn, codedPair, deintValid, decBit, skipCount, outValid)
%#codegen
persistent rIn rDe rOu nIn nDe nOu armIn skp;
if isempty(rIn)
  rIn=uint32(0); rDe=uint32(0); rOu=uint32(0);
  nIn=uint16(0); nDe=uint16(0); nOu=uint16(0); armIn=false; skp=uint16(0);
end
% sync-semantics compliant (RXROOT E11c): locals, persist last.
a=rIn; b=rDe; c=rOu; xIn=nIn; xDe=nDe; xOu=nOu; arm=armIn; sk=skp; %#ok<NASGU>
% --- CAP_IN: first 32 coded-in bits, armed at startIn, gated by validIn ---
if validIn
  if startIn, xIn=uint16(0); a=uint32(0); arm=true; end
  if arm && xIn < uint16(32)
    if bitsIn, a = bitor(a, bitshift(uint32(1), double(xIn))); end
    xIn = xIn + uint16(1);
  end
end
% --- CAP_DEINT: first 32 deint-output coded bits (2 per pair), gated by deintValid ---
if startIn, xDe=uint16(0); b=uint32(0); end
if deintValid && xDe < uint16(32)
  b0 = codedPair(1) ~= 0; b1 = codedPair(2) ~= 0;
  if b0, b = bitor(b, bitshift(uint32(1), double(xDe))); end
  xDe = xDe + uint16(1);
  if xDe < uint16(32)
    if b1, b = bitor(b, bitshift(uint32(1), double(xDe))); end
    xDe = xDe + uint16(1);
  end
end
% --- CAP_OUT (RXROOT E8): first 32 bits of the WRAPPER OUTPUT stream ---
% i6 = RxAlign dataOut gated by i8 = RxAlign validOut: exactly the bits the
% BIST compares, alignment-independent. Golden expectation 0x04922282.
sc = uint16(skipCount); sk = uint16(0); %#ok<NASGU>
if startIn, xOu=uint16(0); c=uint32(0); end
if outValid && xOu < uint16(32)
  if decBit, c = bitor(c, bitshift(uint32(1), double(xOu))); end
  xOu = xOu + uint16(1);
end
capIn = a; capDeint = b; capOut = c;
rIn=a; rDe=b; rOu=c; nIn=xIn; nDe=xDe; nOu=xOu; armIn=arm; skp=sk;

== matlab function commhdlQPSKTxRxLoopback/TxRxComposite/Receiver/QPSK Rx/FecCaptureCadence ==
  data: startIn input; capCad output; validIn input
function capCad = fecCaptureCadence(startIn, validIn)
%#codegen
persistent sCnt gap snv vrun seenStart sawValid measuring;
if isempty(sCnt)
  sCnt=uint8(0); gap=uint8(0); snv=uint8(0); vrun=uint8(0);
  seenStart=false; sawValid=false; measuring=false;
end
% sync-semantics compliant (RXROOT E11c): locals, persist last.
sC=sCnt; gp=gap; sv=snv; vr=vrun; seen=seenStart; saw=sawValid; mea=measuring;
if startIn
  if sC < uint8(255), sC = sC + uint8(1); end
  if ~validIn && sv < uint8(255), sv = sv + uint8(1); end
  if ~seen
    seen = true; mea = true; gp = uint8(0); saw=false; vr=uint8(0);
  end
end
if mea && ~saw
  if validIn
    saw = true;
  elseif gp < uint8(255)
    gp = gp + uint8(1);
  end
end
if seen && validIn && vr < uint8(255)
  vr = vr + uint8(1);
end
capCad = bitor(bitor(uint32(sC), bitshift(uint32(gp),8)), bitor(bitshift(uint32(sv),16), bitshift(uint32(vr),24)));
sCnt=sC; gap=gp; snv=sv; vrun=vr; seenStart=seen; sawValid=saw; measuring=mea;

== matlab function commhdlQPSKTxRxLoopback/TxRxComposite/Receiver/QPSK Rx/RstCsCounter ==
  data: e input; c output
function c = rstCsCount(e)
%#codegen
% Count RISING EDGES of the CFO-step-detector carrier-sync reset (AXI 0x150).
% Saturating; reset by the modem soft-reset 0x000 via the persistent init.
persistent prev cnt;
if isempty(prev), prev = false; cnt = uint32(0); end
n = cnt;
if e && ~prev && n < uint32(4294967295)
    n = n + uint32(1);
end
c = n;
cnt = n;
prev = logical(e);

== matlab function commhdlQPSKTxRxLoopback/TxRxComposite/AdcForensic ==
  data: v input; y output; dI input
function y = adcForensic(v, dI)
%#codegen
% T8.3 ingest forensic (AXI 0x15C): [validDuty|maxGap|maxBurst|levelLog].
% Full-clk-rate; cleared by modem soft-reset 0x000 via persistent init.
persistent wcnt vcnt duty gapc maxGap burc maxBur mx
if isempty(wcnt)
    wcnt = uint16(0); vcnt = uint16(0); duty = uint8(0);
    gapc = uint8(0); maxGap = uint8(0); burc = uint8(0); maxBur = uint8(0);
    mx = uint16(0);
end
w = wcnt; vc = vcnt; d = duty; g = gapc; mg = maxGap;
b = burc; mb = maxBur; m = mx;
if v
    vc = vc + uint16(1);
    if b < uint8(255), b = b + uint8(1); end
    if b > mb, mb = b; end
    g = uint8(0);
    a = uint16(min(abs(int32(dI)), int32(32767)));
    if a > m, m = a; end
else
    if g < uint8(255), g = g + uint8(1); end
    if g > mg, mg = g; end
    b = uint8(0);
end
w = w + uint16(1);
if w >= uint16(8192)
    d = uint8(min(bitshift(vc, -5), uint16(255)));
    w = uint16(0); vc = uint16(0);
end
lv = uint8(0);
for k = 0:15
    if bitshift(m, -k) ~= uint16(0)
        lv = uint8(k + 1);
    end
end
y = bitor(bitor(uint32(d), bitshift(uint32(mg), 8)), ...
          bitor(bitshift(uint32(mb), 16), bitshift(uint32(lv), 24)));
wcnt = w; vcnt = vc; duty = d; gapc = g; maxGap = mg;
burc = b; maxBur = mb; mx = m;

== matlab function commhdlQPSKTxRxLoopback/TxRxComposite/Receiver/QPSK Rx/StatePairProbe ==
  data: uAgcIn input; agcIn output; uAgcOut input; uCsIn input; uCsOut input; agcOut output; csIn output; csOut output
function [agcIn, agcOut, csIn, csOut] = statePairProbe(uAgcIn, uAgcOut, uCsIn, uCsOut)
%#codegen
persistent rAI rAO rCI rCO cnt;
if isempty(rAI)
  rAI=uint32(0); rAO=uint32(0); rCI=uint32(0); rCO=uint32(0); cnt=uint16(0);
end
a=rAI; b=rAO; c=rCI; d=rCO; n=cnt;
if n == uint16(0)
  a = pack_iq(uAgcIn); b = pack_iq(uAgcOut);
  c = pack_iq(uCsIn);  d = pack_iq(uCsOut);
end
n = n + uint16(1);
if n >= uint16(4096), n = uint16(0); end
agcIn = a; agcOut = b; csIn = c; csOut = d;
rAI=a; rAO=b; rCI=c; rCO=d; cnt=n;
end
function p = pack_iq(u)
ri = reinterpretcast(real(u), numerictype(0,16,0));
qi = reinterpretcast(imag(u), numerictype(0,16,0));
p = bitor(bitshift(uint32(ri), 16), uint32(qi));
end

== matlab function commhdlQPSKTxRxLoopback/TxRxComposite/Receiver/QPSK Rx/Frequency and Time Synchronizer/Symbol Synchronizer/ShadowScore ==
  data: pP input; pdivCnt output; pS input; iP input; iS input; und input; pdivBeat output; idivBeat output; ipLatch output; isLatch output; strobeFor output; beatCnt output
function [pdivCnt,pdivBeat,idivBeat,ipLatch,isLatch,strobeFor,beatCnt] = shadowScore(pP,pS,iP,iS,und)
%#codegen
persistent pc pb ib ipl isl mg mingap gap bt pmPrev
if isempty(pc)
  pc=uint32(0); pb=uint32(0); ib=uint32(0); ipl=uint32(0); isl=uint32(0);
  mg=uint16(0); mingap=uint16(65535); gap=uint16(0); bt=uint32(0); pmPrev=false;
end
bt = bt + uint32(1);
% P-path upset events (FIR memory self-heals -> every upset = one edge)
pm = (pP ~= pS);
if pm && ~pmPrev
  pc = pc + uint32(1); pb = bt;
end
pmPrev = pm;
% first integrator divergence: latch beat + both raw state words
if ib == uint32(0) && (iP ~= iS)
  ib = bt;
  ipl = uint32(reinterpretcast(iP, numerictype(0,30,0)));
  isl = uint32(reinterpretcast(iS, numerictype(0,30,0)));
end
% symbol-strobe forensic (nominal Underflow spacing 8 beats; >12 = skip)
if gap < uint16(65535), gap = gap + uint16(1); end
if und
  if gap > mg, mg = gap; end
  if gap < mingap, mingap = gap; end
  gap = uint16(0);
end
pdivCnt = pc; pdivBeat = pb; idivBeat = ib; ipLatch = ipl; isLatch = isl;
strobeFor = bitor(bitshift(uint32(mg),16), uint32(mingap));
beatCnt = bt;

== matlab function commhdlQPSKTxRxLoopback/TxRxComposite/CanaryLfsr ==
  data: x output
function x = canaryLfsr()
%#codegen
persistent s
if isempty(s), s = uint32(2463534242); end
x = s;
s = bitxor(s, bitshift(s, 13));
s = bitxor(s, bitshift(s, -17));
s = bitand(bitxor(s, bitshift(s, 5)), uint32(4294967295));
